simulink model "amplifierboard"  (R2020b)
settings: Solver=FixedStepDiscrete  StartTime=0.0  StopTime=2  FixedStep=0.01  RelTol=1e-3
InitFcn:
  | mbd_s32k_consistency_checks(bdroot(gcs));
undefined symbols (not defined in the file): AutoLowerVal, AutoRaiseVal, HoldVal, LED_En, LED_Off, LED_On, Logic_High, Logic_Low, LQFP, ManualLowerVal, ManualRaiseVal, PWRWNDW_CHDLCK, sC_bool_PWMEN, sC_cnt_FWSetting, sC_cnt_Mtr_DrvNo_HB, sC_cnt_PWMHB1to4, sC_cnt_PWMHB5to8, sC_cnt_TargetSlowRange, sC_pct_ManualMax, sC_pct_RampDwn, sC_pct_RampUp, sC_pct_StartPWM, sC_pct_Targetmax, SwitchPackRangeOffset, Threshold_Value, Tolerant_Time
libraries: mbd_s32k1xx_ec_toolbox x205, simulink x59, canmsglib x19, Filter x15, wndwcmd x3
(part 1 of 6)
settings Model: Creator=ur013317  LastModifiedBy=paulstu3
settings DataIOCC: ExternalInput=off  InitialState=off  SaveOutput=off  SignalLogging=off  SaveTime=off
settings OptimizationCC: DefaultParameterBehavior=Inlined  StrengthReduction=on  PassReuseOutputArgsAs=Individual arguments  ZeroExternalMemoryAtStartup=off  ZeroInternalMemoryAtStartup=off  OptimizeBlockOrder=speed  OptimizationPriority=Speed  OptimizationCustomize=off  MultiThreadedLoops=on  EfficientTunableParamExpr=on
settings DebuggingCC: InheritedTsInSrcMsg=none  SingleTaskRateTransMsg=error  ParameterTunabilityLossMsg=error  UnconnectedInputMsg=error  UnconnectedOutputMsg=error  UnconnectedLineMsg=error  UnknownTsInhSupMsg=error
settings HardwareCC: ProdBitPerPointer=32  ProdBitPerSizeT=32  ProdBitPerPtrDiffT=32  ProdLargestAtomicInteger=Long  ProdLargestAtomicFloat=Double  ProdWordSize=32  ProdHWDeviceType=ARM Compatible->ARM Cortex
settings SFSimCC: MATLABDynamicMemAlloc=off
settings RTWCC: Description=Model Based Design Toolbox S32K1xx Code Generation Target  SystemTargetFile=mbd_s32k.tlc  MakeCommand=mbd_s32k_make_rtw COPY_MDLREF_INCLUDES=0  TemplateMakefile=mbd_s32k.tmf  GenerateReport=on  IncludeHyperlinkInReport=on  LaunchReport=on  GenerateTraceInfo=on  GenerateTraceReport=on  GenerateTraceReportSl=on  GenerateTraceReportSf=on  GenerateTraceReportEml=on  CheckMdlBeforeBuild=Warning
settings CodeAppCC: ForceParamTrailComments=on  IgnoreCustomStorageClasses=off  OperatorAnnotations=on  SimulinkDataObjDesc=on  SFDataObjDesc=on  InsertBlockDesc=on
settings STFCustomTargetCC: TargetLangStandard=C99 (ISO)  MultiwordLength=256  ConcurrentExecutionCompliant=off  CombineOutputUpdateFcns=on  ERTCustomFileBanners=on  SupportContinuousTime=off  SupportNonInlinedSFcns=off  RemoveResetFunc=on  MATLABClassNameForMDSCustomization=Simulink.SoftwareTarget.ERTCustomization  CPPClassGenCompliant=off  GRTInterface=off  SystemTargetFile=mbd_s32k.tlc
settings ERTTargetCC: TargetLangStandard=C99 (ISO)  ParMdlRefBuildCompliant=off  CompOptLevelCompliant=off  ConcurrentExecutionCompliant=off  ModelStepFunctionPrototypeControlCompliant=off  CPPClassGenCompliant=off  UseToolchainInfoCompliant=off  InlinedParameterPlacement=NonHierarchical  ERTSrcFileBannerTemplate=mbd_ert_code_template.cgt  ERTHdrFileBannerTemplate=mbd_ert_code_template.cgt  ERTDataSrcFileTemplate=mbd_ert_code_template.cgt  ERTDataHdrFileTemplate=mbd_ert_code_template.cgt  ERTCustomFileTemplate=example_file_process.tlc

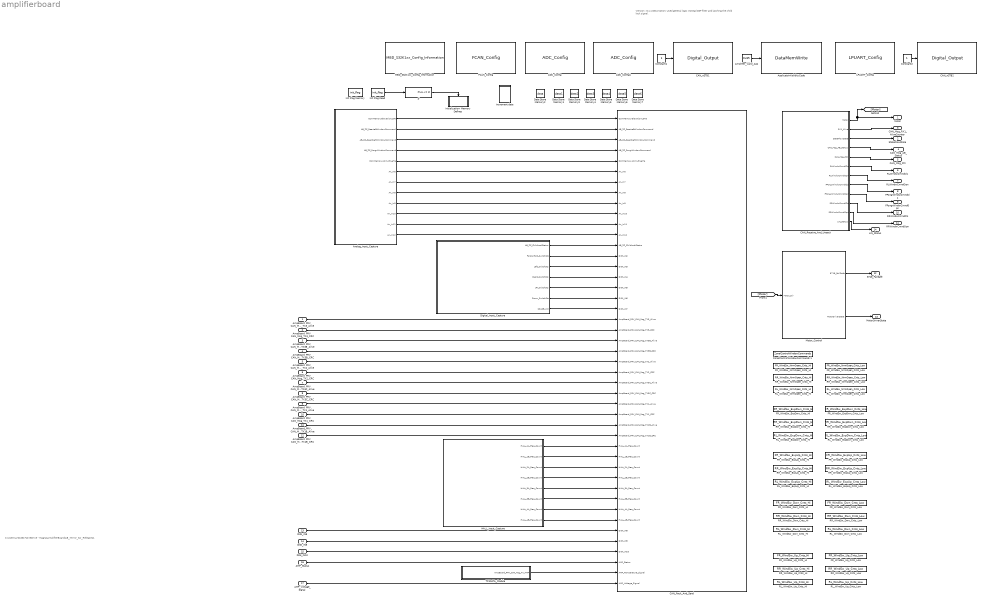
== system amplifierboard ==
  note: C:\Users\ur013317\OneDrive - Magna\AmplifierBoard\AB_Mirror_Sw_Release11
  note: Version : 6.1.1
      | Description:
      | Used general logic instead DSP filter and latching the child lock signal.
  AmpBoard_PRV_CAN_Msg_TX3_Alive : Inport
  AmpBoard_PRV_CAN_Msg_TX3_CRC : Inport  Port=2
  AmpBoard_PRV_CAN_Msg_TX3B_Alive : Inport  Port=3
  AmpBoard_PRV_CAN_Msg_TX3B_CRC : Inport  Port=4
  AmpBoard_PRV_CAN_Msg_TX2_Alive : Inport  Port=5
  AmpBoard_PRV_CAN_Msg_TX2_CRC : Inport  Port=6
  AmpBoard_PRV_CAN_Msg_TX3C_Alive : Inport  Port=7
  AmpBoard_PRV_CAN_Msg_TX3C_CRC : Inport  Port=8
  AmpBoard_PRV_CAN_Msg_TX1_Alive : Inport  Port=9
  AmpBoard_PRV_CAN_Msg_TX1_CRC : Inport  Port=10
  AmpBoard_PRV_CAN_Msg_TX1B_Alive : Inport  Port=11
  AmpBoard_PRV_CAN_Msg_TX1B_CRC : Inport  Port=12
  DIGI_IN8 : Inport  Port=13
  DIGI_IN9 : Inport  Port=14
  DIGI_IN10 : Inport  Port=15
  AMP_Status : Inport  Port=16
  AMP_Voltage_SIgnal : Inport  Port=17
  ADC_Config : mbd_s32k1xx_ec_toolbox/Motor Control Blocks/ADC Blocks/ADC_Config  instance=1  mode=12-bit conversion  smplts=2  adiclk=alternate clock 1  adiv=input clock  show_adv_opts=off  pretrgsel=PDB pre-trigger  swpretrg=Disabled  adtrg=software  trgsel=TRGMUX output  refsel=Vrefh and Vrefl  supply_monitoring=off  acfe=off  acfgt=off  acren=off  cv1=0  cv2=0  adco=off  avge=off  avgs=4 samples
  ADC_Config1 : mbd_s32k1xx_ec_toolbox/Motor Control Blocks/ADC Blocks/ADC_Config  instance=0  mode=12-bit conversion  smplts=2  adiclk=alternate clock 1  adiv=input clock  show_adv_opts=off  pretrgsel=PDB pre-trigger  swpretrg=Disabled  adtrg=software  trgsel=TRGMUX output  refsel=Vrefh and Vrefl  supply_monitoring=off  acfe=off  acfgt=off  acren=off  cv1=0  cv2=0  adco=off  avge=off  avgs=4 samples
  Amplifier_Valid_App : Constant  Value=0x85  OutDataTypeStr=uint8
  Analog_Input_Capture : Subsystem
  ApplicatoinValidityCode : mbd_s32k1xx_ec_toolbox/Utility Blocks/DataMemWrite  Priority=15  base=0x14000000  offset=0x0000  ptr=uint8_t
  CAN_Pack_And_Send : Subsystem
  CAN_Receive_And_Unpack : Subsystem
  CAN_nSTB1 : mbd_s32k1xx_ec_toolbox/GPIO Blocks/Digital_Output  gpio_pin=PTE3: [PTE3 | Port E I/O]  init_val=High  drive_strength=High
  CAN_nSTB2 : mbd_s32k1xx_ec_toolbox/GPIO Blocks/Digital_Output  gpio_pin=PTD11: [PTD11 | Port D I/O]  init_val=High  drive_strength=High
  Constant1 : Constant  OutDataTypeStr=boolean
  Constant2 : Constant  OutDataTypeStr=boolean
  Data Store Memory1 : DataStoreMemory  DataStoreName=data1  ReadBeforeWriteMsg=warning  WriteAfterWriteMsg=warning  WriteAfterReadMsg=warning  ShowAdditionalParam=off
  Data Store Memory2 : DataStoreMemory  DataStoreName=data  ReadBeforeWriteMsg=warning  WriteAfterWriteMsg=warning  WriteAfterReadMsg=warning  ShowAdditionalParam=off
  Data Store Memory3 : DataStoreMemory  DataStoreName=data2  ReadBeforeWriteMsg=warning  WriteAfterWriteMsg=warning  WriteAfterReadMsg=warning  ShowAdditionalParam=off
  Data Store Memory4 : DataStoreMemory  DataStoreName=data3  ReadBeforeWriteMsg=warning  WriteAfterWriteMsg=warning  WriteAfterReadMsg=warning  ShowAdditionalParam=off
  Data Store Memory5 : DataStoreMemory  DataStoreName=data4  ReadBeforeWriteMsg=warning  WriteAfterWriteMsg=warning  WriteAfterReadMsg=warning  ShowAdditionalParam=off
  Data Store Memory6 : DataStoreMemory  DataStoreName=data5  ReadBeforeWriteMsg=warning  WriteAfterWriteMsg=warning  WriteAfterReadMsg=warning  ShowAdditionalParam=off
  Data Store Memory7 : DataStoreMemory  DataStoreName=data6  ReadBeforeWriteMsg=warning  WriteAfterWriteMsg=warning  WriteAfterReadMsg=warning  ShowAdditionalParam=off
  Digital_Input_Capture : Subsystem
  FCAN_Config : mbd_s32k1xx_ec_toolbox/Communication Blocks/CAN Blocks/FCAN_Config  Priority=1  can_instance=1  can_mode=Normal mode  can_max_num_mb=32  can_rx=PTC6: [CAN1_RX | CAN Rx channel]  can_tx=PTC7: [CAN1_TX | CAN Tx Channel]  show_adv_opts=on  can_clk_src=Peripheral clock  can_clk_freq=80 MHz  bitrate_to_time_seg=on  bitrate=500  sample_point=87.5  real_bitrate=500  real_sample_point=87.5  prop_delay=250  bus_length=1  tq=125.0  time_quanta=16  can_presdiv=10  can_propseg=5  can_pseg1=8  can_pseg2=2  can_rjw=2  cbt_bitrate=2000  cbt_sample_point=80  cbt_real_bitrate=2000  cbt_real_sample_point=80  cbt_tq=25.0  cbt_time_quanta=40  can_cbt_presdiv=4  can_cbt_propseg=9  can_cbt_pseg1=5  can_cbt_pseg2=5  can_cbt_rjw=3  can_fd_enable=off  can_payload=8  tdc_enable=off  tdc_offset=20  can_rxfifo_enable=off  can_num_id_filters=8  can_fifo_id_format=A  can_fifo_id_filter={{false,false,'0x2'},{false,false,'0x3'},{false,false,'0x4'},{false,false,'0xAB'},{false,false,'0x0'},{false,false,'0x0'},{false,false,'0x0'},{false,false,'0x0'}}  can_pn_enable=off  can_wakeup_match=off  can_wakeup_timeout=off  can_timeout_en=off  can_match_timeout=1  can_multiple_matches_en=off  can_num_matches=1  can_idfilter_extendedid=off  can_idfilter_remoteframe=off  can_idfilter_type=Match exact  can_idfilter_id1=0  can_idfilter_id2=0  can_payloadfilter_enable=off  can_payloadfilter_dlclow=0  can_payloadfilter_dlchigh=0  can_payloadfilter_type=Match exact  can_payloadfilter_payload1_b0=0  can_payloadfilter_payload1_b1=0  can_payloadfilter_payload1_b2=0  can_payloadfilter_payload1_b3=0  can_payloadfilter_payload1_b4=0  can_payloadfilter_payload1_b5=0  can_payloadfilter_payload1_b6=0  can_payloadfilter_payload1_b7=0  can_payloadfilter_payload2_b0=0  can_payloadfilter_payload2_b1=0  can_payloadfilter_payload2_b2=0  can_payloadfilter_payload2_b3=0  can_payloadfilter_payload2_b4=0  can_payloadfilter_payload2_b5=0  can_payloadfilter_payload2_b6=0  can_payloadfilter_payload2_b7=0
  FR_WindSw_Dwn_Cnts_Hi : DataStoreMemory  DataStoreName=FR_WindSw_Dwn_Cnts_Hi  ReadBeforeWriteMsg=warning  WriteAfterWriteMsg=warning  WriteAfterReadMsg=warning  ShowAdditionalParam=off  OutDataTypeStr=uint16
  FR_WindSw_Dwn_Cnts_Low : DataStoreMemory  DataStoreName=FR_WindSw_Dwn_Cnts_Low  ReadBeforeWriteMsg=warning  WriteAfterWriteMsg=warning  WriteAfterReadMsg=warning  ShowAdditionalParam=off  OutDataTypeStr=uint16
  FR_WindSw_ExpDwn_Cnts_Hi : DataStoreMemory  DataStoreName=FR_WindSw_ExpDwn_Cnts_Hi  ReadBeforeWriteMsg=warning  WriteAfterWriteMsg=warning  WriteAfterReadMsg=warning  ShowAdditionalParam=off  OutDataTypeStr=uint16
  FR_WindSw_ExpDwn_Cnts_Low : DataStoreMemory  DataStoreName=FR_WindSw_ExpDwn_Cnts_Low  ReadBeforeWriteMsg=warning  WriteAfterWriteMsg=warning  WriteAfterReadMsg=warning  ShowAdditionalParam=off  OutDataTypeStr=uint16
  FR_WindSw_ExpUp_Cnts_Hi : DataStoreMemory  DataStoreName=FR_WindSw_ExpUp_Cnts_Hi  ReadBeforeWriteMsg=warning  WriteAfterWriteMsg=warning  WriteAfterReadMsg=warning  ShowAdditionalParam=off  OutDataTypeStr=uint16
  FR_WindSw_ExpUp_Cnts_Low : DataStoreMemory  DataStoreName=FR_WindSw_ExpUp_Cnts_Low  ReadBeforeWriteMsg=warning  WriteAfterWriteMsg=warning  WriteAfterReadMsg=warning  ShowAdditionalParam=off  OutDataTypeStr=uint16
  "FR_WindSw_NrmOpen_Cnts_Hi " : DataStoreMemory  DataStoreName=FR_WindSw_NrmOpen_Cnts_Hi  ReadBeforeWriteMsg=warning  WriteAfterWriteMsg=warning  WriteAfterReadMsg=warning  ShowAdditionalParam=off  OutDataTypeStr=uint16
  FR_WindSw_NrmOpen_Cnts_Low : DataStoreMemory  DataStoreName=FR_WindSw_NrmOpen_Cnts_Low  ReadBeforeWriteMsg=warning  WriteAfterWriteMsg=warning  WriteAfterReadMsg=warning  ShowAdditionalParam=off  OutDataTypeStr=uint16
  FR_WindSw_Up_Cnts_Hi : DataStoreMemory  DataStoreName=FR_WindSw_Up_Cnts_Hi  ReadBeforeWriteMsg=warning  WriteAfterWriteMsg=warning  WriteAfterReadMsg=warning  ShowAdditionalParam=off  OutDataTypeStr=uint16
      settings: LockScale=on
  FR_WindSw_Up_Cnts_Low : DataStoreMemory  DataStoreName=FR_WindSw_Up_Cnts_Low  ReadBeforeWriteMsg=warning  WriteAfterWriteMsg=warning  WriteAfterReadMsg=warning  ShowAdditionalParam=off  OutDataTypeStr=uint16
  HALL_Input_Capture : Subsystem
  If : If  IfExpression=u1 <= 2  ShowElse=off
  Increment data : Subsystem
  Init Flag Memory : DataStoreMemory  DataStoreName=init_flag  ReadBeforeWriteMsg=warning  WriteAfterWriteMsg=warning  WriteAfterReadMsg=warning  ShowAdditionalParam=off  OutDataTypeStr=fixdt('uint8', 'DataTypeOverride', 'Off')
  Init Flag Read : DataStoreRead  DataStoreName=init_flag  DataStoreElements=init_flag
  Initialization- Memory Defines : Subsystem  TreatAsAtomicUnit=on
  LPUART_Config : mbd_s32k1xx_ec_toolbox/Communication Blocks/UART Blocks/LPUART_Config  instance=2  baudrate=115200  custom_baudrate=1000000  databits=8  parity=None  sbns=1  bothedge=rising edge  rxinv=off  txinv=off  show_adv_opts=off  brk13=10 - 13 bit times  lbkde=10 - 13 bit times  rx=PTD6: [LPUART2_RX | Receive]  tx=PTD7: [LPUART2_TX | Transmit]
  MBD_S32K1xx_Config_Information : mbd_s32k1xx_ec_toolbox/MBD_S32K1xx_Config_Information  Priority=2  mbdt_ver=0  disp_str=|  config_params=[]  mcu_target_name=S32K146  mcu_target_package=100-LQFP  mcu_target_sram_size=128KB  mcu_system_clock_freq=80  mcu_xtal_freq=External 40  mcu_steptick_timer=LPIT Channel 0  mcu_steptick_prio=15  ds_import_enable=on  target_compiler=GCC  target_memory=FLASH  gcc_target_compile_opts=-mthumb -mfloat-abi=hard -mfpu=fpv4-sp-d16 -O1 -g -gstrict-dwarf  gcc_target_assemble_opts=-mthumb -mfloat-abi=hard -mfpu=fpv4-sp-d16 -g  gcc_target_link_opts=-mthumb -mfloat-abi=hard -mfpu=fpv4-sp-d16  gcc_target_default_lcf=off  gcc_target_user_lcf=S32K146_128_flash.ld  ghs_target_compile_opts=-cpu=cortexm4f -thumb -fpu=vfpv4_d16 -fsingle -Ogeneral -Wundef -Wimplicit-int -Wshadow -Wtrigraphs --no_commons --gnu_asm -gnu99 -gdwarf-2 -G  ghs_target_assemble_opts=-cpu=cortexm4f -fpu=vfpv4_d16  ghs_target_link_opts=-cpu=cortexm4f -thumb -fpu=vfpv4_d16  ghs_target_default_lcf=on  ghs_target_user_lcf=S32K146_128_flash.ld  iar_target_compile_opts=--cpu=Cortex-M4F --thumb --fpu=VFPv4_sp -Ol -e --debug --dlib_config normal  iar_target_assemble_opts=--cpu Cortex-M4F --thumb --fpu VFPv4_sp  iar_target_link_opts=--no_exceptions --vfe --inline  iar_target_default_lcf=on  iar_target_user_lcf=S32K146_128_flash.icf  pil_download_enable=off  rbl_download_enable=on  rbl_start_delay=5000  rbl_download_interface=OpenSDA  rbl_restart_request=off  rbl_com_port=Custom  rbl_com_port_custom=COM1  pil_download_rate=57600  pil_download_rate_custom=115200  pil_opensda_drive=Custom  pil_opensda_drive_custom=D  jtag_interface=OpenSDA Embedded Debug  jlink_default_path=on  jlink_user_path=C:\Program Files\SEGGER\JLink\  pil_uart_instance=1  pil_uart_rx=PTC6: [LPUART1_RX | Receive]  pil_uart_tx=PTC7: [LPUART1_TX | Transmit]  FTM_PWM_PcrCheckEnDis=on  FTM_Input_Edge_Inputs_PcrCheckEnDis=on  FTM_Dual_Edge_Inputs_PcrCheckEnDis=on  FTM_Quadrature_Inputs_PcrCheckEnDis=on  FTM_Hall_Sensor_Inputs_PcrCheckEnDis=on  LPTMR_PcrCheckEnDis=on  PIT_PcrCheckEnDis=on  RTC_PcrCheckEnDis=on  FlexCAN_PcrCheckEnDis=on  LIN_PcrCheckEnDis=on  FlexIO_PcrCheckEnDis=on  LPI2C_PcrCheckEnDis=on  LPSPI_PcrCheckEnDis=on  LPUART_PcrCheckEnDis=on  CMP_PcrCheckEnDis=on  GPIO_OutputPcrCheckEnDis=on  GPIO_InputPcrCheckEnDis=on  SBC_PcrCheckEnDis=on  BMS_PcrCheckEnDis=on  AMMCLIB_PcrCheckEnDis=on  FM_PcrCheckEnDis=on  Profile_PcrCheckEnDis=on  ConfigParams_PcrCheckEnDis=on  ModelRef_PcrCheckEnDis=on  PDB0_PcrCheckEnDis=on  CSEc_PcrCheckEnDis=on  eDMA_PcrCheckEnDis=on  FLASH_PcrCheckEnDis=on  ADC_PcrCheckEnDis=on  WDOG_PcrCheckEnDis=on
      | Target : S32K144-64KB_SRAM
      | Package : 100-pin
      | System clock : 80 MHz
      | XTAL clock : External 8 MHz
      | Compiler : IAR
      | Target Type : FLASH
      | Download Code after build : off
      | Step Tick Interrupt Priority : 15
  Motor_Control : Subsystem
  RL_WindSw_Dwn_Cnts_Hi : DataStoreMemory  DataStoreName=RL_WindSw_Dwn_Cnts_Hi  ReadBeforeWriteMsg=warning  WriteAfterWriteMsg=warning  WriteAfterReadMsg=warning  ShowAdditionalParam=off  OutDataTypeStr=uint16
  RL_WindSw_Dwn_Cnts_Low : DataStoreMemory  DataStoreName=RL_WindSw_Dwn_Cnts_Low  ReadBeforeWriteMsg=warning  WriteAfterWriteMsg=warning  WriteAfterReadMsg=warning  ShowAdditionalParam=off  OutDataTypeStr=uint16
  RL_WindSw_ExpDwn_Cnts_Hi : DataStoreMemory  DataStoreName=RL_WindSw_ExpDwn_Cnts_Hi  ReadBeforeWriteMsg=warning  WriteAfterWriteMsg=warning  WriteAfterReadMsg=warning  ShowAdditionalParam=off  OutDataTypeStr=uint16
  RL_WindSw_ExpDwn_Cnts_Low : DataStoreMemory  DataStoreName=RL_WindSw_ExpDwn_Cnts_Low  ReadBeforeWriteMsg=warning  WriteAfterWriteMsg=warning  WriteAfterReadMsg=warning  ShowAdditionalParam=off  OutDataTypeStr=uint16
  RL_WindSw_ExpUp_Cnts_Hi : DataStoreMemory  DataStoreName=RL_WindSw_ExpUp_Cnts_Hi  ReadBeforeWriteMsg=warning  WriteAfterWriteMsg=warning  WriteAfterReadMsg=warning  ShowAdditionalParam=off  OutDataTypeStr=uint16
  RL_WindSw_ExpUp_Cnts_Low : DataStoreMemory  DataStoreName=RL_WindSw_ExpUp_Cnts_Low  ReadBeforeWriteMsg=warning  WriteAfterWriteMsg=warning  WriteAfterReadMsg=warning  ShowAdditionalParam=off  OutDataTypeStr=uint16
  RL_WindSw_NrmOpen_Cnts_Hi : DataStoreMemory  DataStoreName=RL_WindSw_NrmOpen_Cnts_Hi  ReadBeforeWriteMsg=warning  WriteAfterWriteMsg=warning  WriteAfterReadMsg=warning  ShowAdditionalParam=off  OutDataTypeStr=uint16
  RL_WindSw_NrmOpen_Cnts_Low : DataStoreMemory  DataStoreName=RL_WindSw_NrmOpen_Cnts_Low  ReadBeforeWriteMsg=warning  WriteAfterWriteMsg=warning  WriteAfterReadMsg=warning  ShowAdditionalParam=off  OutDataTypeStr=uint16
  RL_WindSw_Up_Cnts_Hi : DataStoreMemory  DataStoreName=RL_WindSw_Up_Cnts_Hi  ReadBeforeWriteMsg=warning  WriteAfterWriteMsg=warning  WriteAfterReadMsg=warning  ShowAdditionalParam=off  OutDataTypeStr=uint16
  RL_WindSw_Up_Cnts_Low : DataStoreMemory  DataStoreName=RL_WindSw_Up_Cnts_Low  ReadBeforeWriteMsg=warning  WriteAfterWriteMsg=warning  WriteAfterReadMsg=warning  ShowAdditionalParam=off  OutDataTypeStr=uint16
  RR_WindSw_Dwn_Cnts_Hi : DataStoreMemory  DataStoreName=RR_WindSw_Dwn_Cnts_Hi  ReadBeforeWriteMsg=warning  WriteAfterWriteMsg=warning  WriteAfterReadMsg=warning  ShowAdditionalParam=off  OutDataTypeStr=uint16
  RR_WindSw_Dwn_Cnts_Low : DataStoreMemory  DataStoreName=RR_WindSw_Dwn_Cnts_Low  ReadBeforeWriteMsg=warning  WriteAfterWriteMsg=warning  WriteAfterReadMsg=warning  ShowAdditionalParam=off  OutDataTypeStr=uint16
  RR_WindSw_ExpDwn_Cnts_Hi : DataStoreMemory  DataStoreName=RR_WindSw_ExpDwn_Cnts_Hi  ReadBeforeWriteMsg=warning  WriteAfterWriteMsg=warning  WriteAfterReadMsg=warning  ShowAdditionalParam=off  OutDataTypeStr=uint16
  RR_WindSw_ExpDwn_Cnts_Low : DataStoreMemory  DataStoreName=RR_WindSw_ExpDwn_Cnts_Low  ReadBeforeWriteMsg=warning  WriteAfterWriteMsg=warning  WriteAfterReadMsg=warning  ShowAdditionalParam=off  OutDataTypeStr=uint16
  RR_WindSw_ExpUp_Cnts_Hi : DataStoreMemory  DataStoreName=RR_WindSw_ExpUp_Cnts_Hi  ReadBeforeWriteMsg=warning  WriteAfterWriteMsg=warning  WriteAfterReadMsg=warning  ShowAdditionalParam=off  OutDataTypeStr=uint16
  RR_WindSw_ExpUp_Cnts_Low : DataStoreMemory  DataStoreName=RR_WindSw_ExpUp_Cnts_Low  ReadBeforeWriteMsg=warning  WriteAfterWriteMsg=warning  WriteAfterReadMsg=warning  ShowAdditionalParam=off  OutDataTypeStr=uint16
  RR_WindSw_NrmOpen_Cnts_Hi : DataStoreMemory  DataStoreName=RR_WindSw_NrmOpen_Cnts_Hi  ReadBeforeWriteMsg=warning  WriteAfterWriteMsg=warning  WriteAfterReadMsg=warning  ShowAdditionalParam=off  OutDataTypeStr=uint16
  RR_WindSw_NrmOpen_Cnts_Low : DataStoreMemory  DataStoreName=RR_WindSw_NrmOpen_Cnts_Low  ReadBeforeWriteMsg=warning  WriteAfterWriteMsg=warning  WriteAfterReadMsg=warning  ShowAdditionalParam=off  OutDataTypeStr=uint16
  RR_WindSw_Up_Cnts_Hi : DataStoreMemory  DataStoreName=RR_WindSw_Up_Cnts_Hi  ReadBeforeWriteMsg=warning  WriteAfterWriteMsg=warning  WriteAfterReadMsg=warning  ShowAdditionalParam=off  OutDataTypeStr=uint16
  RR_WindSw_Up_Cnts_Low : DataStoreMemory  DataStoreName=RR_WindSw_Up_Cnts_Low  ReadBeforeWriteMsg=warning  WriteAfterWriteMsg=warning  WriteAfterReadMsg=warning  ShowAdditionalParam=off  OutDataTypeStr=uint16
  TC1047A_Module : Subsystem
  ZonalControlWindowCommands 1 : DataStoreMemory  DataStoreName=ZonalControlWindowCommands  ReadBeforeWriteMsg=warning  WriteAfterWriteMsg=warning  WriteAfterReadMsg=warning  ShowAdditionalParam=off  OutDataTypeStr=uint16
  Motor : Outport
  StateFlowState : Outport  Port=2
  CHN_Msg_RX1_AliveCounter : Outport  Port=3
  CAN_Msg_AB_Status : Outport  Port=4
  CAN_Msg_PCI : Outport  Port=5
  RLWindwCmndCls : Outport  Port=6
  RLWindwCmndOpn : Outport  Port=7
  FPsngrWindwCmndCls : Outport  Port=8
  FPsngrWindwCmndOpn : Outport  Port=9
  RRWindwCmndCls : Outport  Port=10
  RRWindwCmndOpn : Outport  Port=11
  8718_FailSafe : Outport  Port=12
  MotorDriverState : Outport  Port=13
  LIN_Status : Outport  Port=14
  wires:
  Constant1/1 -> CAN_nSTB1/1
  If/1 -> Initialization- Memory Defines/Action
  Init Flag Read/1 -> If/1
  [Motor] -> Motor_Control/1(Motor_Dir)
  Analog_Input_Capture/6(An_In6) -> CAN_Pack_And_Send/6(An_In6)
  Analog_Input_Capture/7(An_In7) -> CAN_Pack_And_Send/7(An_In7)
  Analog_Input_Capture/8(An_In8) -> CAN_Pack_And_Send/8(An_In8)
  Analog_Input_Capture/9(An_In9) -> CAN_Pack_And_Send/9(An_In9)
  Analog_Input_Capture/10(An_In10) -> CAN_Pack_And_Send/10(An_In10)
  Analog_Input_Capture/11(An_In11) -> CAN_Pack_And_Send/11(An_In11)
  Analog_Input_Capture/12(An_In12) -> CAN_Pack_And_Send/12(An_In12)
  Digital_Input_Capture/2(FoldUnfold_SwitchSts) -> CAN_Pack_And_Send/14(DIGI_IN2)
  Digital_Input_Capture/3(Left_SwitchSts) -> CAN_Pack_And_Send/15(DIGI_IN3)
  Digital_Input_Capture/4(Right_SwitchSts) -> CAN_Pack_And_Send/16(DIGI_IN4)
  Digital_Input_Capture/5(UP_SwitchSts) -> CAN_Pack_And_Send/17(DIGI_IN5)
  Digital_Input_Capture/6(Down_SwitchSts) -> CAN_Pack_And_Send/18(DIGI_IN6)
  Digital_Input_Capture/7(SPARE_In3) -> CAN_Pack_And_Send/19(DIGI_IN7)
  AmpBoard_PRV_CAN_Msg_TX3_Alive/1 -> CAN_Pack_And_Send/20(AmpBoard_PRV_CAN_Msg_TX3_Alive)
  AmpBoard_PRV_CAN_Msg_TX3_CRC/1 -> CAN_Pack_And_Send/21(AmpBoard_PRV_CAN_Msg_TX3_CRC)
  AmpBoard_PRV_CAN_Msg_TX3B_Alive/1 -> CAN_Pack_And_Send/22(AmpBoard_PRV_CAN_Msg_TX3B_Alive)
  AmpBoard_PRV_CAN_Msg_TX3B_CRC/1 -> CAN_Pack_And_Send/23(AmpBoard_PRV_CAN_Msg_TX3B_CRC)
  AmpBoard_PRV_CAN_Msg_TX2_Alive/1 -> CAN_Pack_And_Send/24(AmpBoard_PRV_CAN_Msg_TX2_Alive)
  AmpBoard_PRV_CAN_Msg_TX2_CRC/1 -> CAN_Pack_And_Send/25(AmpBoard_PRV_CAN_Msg_TX2_CRC)
  AmpBoard_PRV_CAN_Msg_TX3C_Alive/1 -> CAN_Pack_And_Send/26(AmpBoard_PRV_CAN_Msg_TX3C_Alive)
  AmpBoard_PRV_CAN_Msg_TX3C_CRC/1 -> CAN_Pack_And_Send/27(AmpBoard_PRV_CAN_Msg_TX3C_CRC)
  AmpBoard_PRV_CAN_Msg_TX1_Alive/1 -> CAN_Pack_And_Send/28(AmpBoard_PRV_CAN_Msg_TX1_Alive)
  AmpBoard_PRV_CAN_Msg_TX1_CRC/1 -> CAN_Pack_And_Send/29(AmpBoard_PRV_CAN_Msg_TX1_CRC)
  AmpBoard_PRV_CAN_Msg_TX1B_Alive/1 -> CAN_Pack_And_Send/30(AmpBoard_PRV_CAN_Msg_TX1B_Alive)
  AmpBoard_PRV_CAN_Msg_TX1B_CRC/1 -> CAN_Pack_And_Send/31(AmpBoard_PRV_CAN_Msg_TX1B_CRC)
  HALL_Input_Capture/1(HALL_1A_Freq_Count) -> CAN_Pack_And_Send/32(HALL_1A_Freq_Count)
  HALL_Input_Capture/2(HALL_1B_Freq_Count) -> CAN_Pack_And_Send/33(HALL_1B_Freq_Count)
  HALL_Input_Capture/3(HALL_2A_Freq_Count) -> CAN_Pack_And_Send/34(HALL_2A_Freq_Count)
  HALL_Input_Capture/4(HALL_2B_Freq_Count) -> CAN_Pack_And_Send/35(HALL_2B_Freq_Count)
  HALL_Input_Capture/5(HALL_3A_Freq_Count) -> CAN_Pack_And_Send/36(HALL_3A_Freq_Count)
  HALL_Input_Capture/6(HALL_3B_Freq_Count) -> CAN_Pack_And_Send/37(HALL_3B_Freq_Count)
  HALL_Input_Capture/7(HALL_4A_Freq_Count) -> CAN_Pack_And_Send/38(HALL_4A_Freq_Count)
  HALL_Input_Capture/8(HALL_4B_Freq_Count) -> CAN_Pack_And_Send/39(HALL_4B_Freq_Count)
  Analog_Input_Capture/1(OsmMemoryElevationLeHa) -> CAN_Pack_And_Send/1(OsmMemoryElevationLeHa)
  DIGI_IN9/1 -> CAN_Pack_And_Send/41(DIGI_IN9)
  DIGI_IN8/1 -> CAN_Pack_And_Send/40(DIGI_IN8)
  DIGI_IN10/1 -> CAN_Pack_And_Send/42(DIGI_IN10)
  Digital_Input_Capture/1(AB_ZC_ChildLockStatus) -> CAN_Pack_And_Send/13(AB_ZC_ChildLockStatus)
  Analog_Input_Capture/5(OsmMemoryAzimuthLeHa) -> CAN_Pack_And_Send/5(OsmMemoryAzimuthLeHa)
  Analog_Input_Capture/4(AB_ZC_PsngrWindowCommand) -> CAN_Pack_And_Send/4(AB_ZC_PsngrWindowCommand)
  AMP_Voltage_SIgnal/1 -> CAN_Pack_And_Send/45(AMP_Voltage_SIgnal)
  TC1047A_Module/1(AmpBoard_PRV_CAN_Msg_TX_TMP) -> CAN_Pack_And_Send/44(AMP_Temperature_Signal)
  AMP_Status/1 -> CAN_Pack_And_Send/43(AMP_Status)
  Amplifier_Valid_App/1 -> ApplicatoinValidityCode/1
  Analog_Input_Capture/2(AB_ZC_RearLeftWindowCommand) -> CAN_Pack_And_Send/2(AB_ZC_RearLeftWindowCommand)
  Analog_Input_Capture/3(AB_ZC_RearRightWindowCommand) -> CAN_Pack_And_Send/3(AB_ZC_RearRightWindowCommand)
  Constant2/1 -> CAN_nSTB2/1
  CAN_Receive_And_Unpack/11(RRWindwCmndOpn) -> RRWindwCmndOpn/1
  CAN_Receive_And_Unpack/3(StateFlowState) -> StateFlowState/1
  CAN_Receive_And_Unpack/9(FPsngrWindwCmndOpn) -> FPsngrWindwCmndOpn/1
  CAN_Receive_And_Unpack/8(FPsngrWindwCmndCls) -> FPsngrWindwCmndCls/1
  CAN_Receive_And_Unpack/10(RRWindwCmndCls) -> RRWindwCmndCls/1
  CAN_Receive_And_Unpack/7(RLWindwCmndOpn) -> RLWindwCmndOpn/1
  CAN_Receive_And_Unpack/4(CAN_Msg_AB_Status) -> CAN_Msg_AB_Status/1
  CAN_Receive_And_Unpack/2(RX1_Alive) -> CHN_Msg_RX1_AliveCounter/1
  CAN_Receive_And_Unpack/5(CAN_Msg_PCI) -> CAN_Msg_PCI/1
  CAN_Receive_And_Unpack/1(Motor) -> [Motor], Motor/1
  CAN_Receive_And_Unpack/6(RLWindwCmndCls) -> RLWindwCmndCls/1
  Motor_Control/1(8718_FailSafe) -> 8718_FailSafe/1
  Motor_Control/2(MotorDriverState) -> MotorDriverState/1
  CAN_Receive_And_Unpack/12(LIN_Status) -> LIN_Status/1

== system amplifierboard/Analog_Input_Capture ==
  note: Description:- All Analog inputs(12) are captured through ADC block
  AB_ZC_PsngrWindowCommand_In : mbd_s32k1xx_ec_toolbox/Motor Control Blocks/ADC Blocks/ADC_Start  instance=0  adc_r=A  adc_chan=PTB2: [ADC0_SE6 | ADC Single Ended Input]  aien=off  mcuTargetUpdate=on
  AB_ZC_RearLeftWindowCommand_In : mbd_s32k1xx_ec_toolbox/Motor Control Blocks/ADC Blocks/ADC_Start  instance=0  adc_r=A  adc_chan=PTB0: [ADC0_SE4 | ADC Single Ended Input]  aien=off  mcuTargetUpdate=on
  AB_ZC_RearRightWindowCommand_In : mbd_s32k1xx_ec_toolbox/Motor Control Blocks/ADC Blocks/ADC_Start  instance=0  adc_r=A  adc_chan=PTB1: [ADC0_SE5 | ADC Single Ended Input]  aien=off  mcuTargetUpdate=on
  AnIn_1 : mbd_s32k1xx_ec_toolbox/Motor Control Blocks/ADC Blocks/ADC_Start  instance=0  adc_r=A  adc_chan=PTC14: [ADC0_SE12 | ADC Single Ended Input]  aien=off  mcuTargetUpdate=on
  AnIn_10 : mbd_s32k1xx_ec_toolbox/Motor Control Blocks/ADC Blocks/ADC_Start  instance=1  adc_r=A  adc_chan=PTB12: [ADC1_SE7 | ADC Single Ended Input]  aien=off  mcuTargetUpdate=on
  AnIn_11 : mbd_s32k1xx_ec_toolbox/Motor Control Blocks/ADC Blocks/ADC_Start  instance=1  adc_r=A  adc_chan=PTD4: [ADC1_SE6 | ADC Single Ended Input]  aien=off  mcuTargetUpdate=on
  AnIn_12 : mbd_s32k1xx_ec_toolbox/Motor Control Blocks/ADC Blocks/ADC_Start  instance=1  adc_r=A  adc_chan=PTD3: [ADC1_SE3 | ADC Single Ended Input]  aien=off  mcuTargetUpdate=on
  AnIn_5 : mbd_s32k1xx_ec_toolbox/Motor Control Blocks/ADC Blocks/ADC_Start  instance=0  adc_r=A  adc_chan=PTB3: [ADC0_SE7 | ADC Single Ended Input]  aien=off  mcuTargetUpdate=on
  AnIn_6 : mbd_s32k1xx_ec_toolbox/Motor Control Blocks/ADC Blocks/ADC_Start  instance=0  adc_r=A  adc_chan=PTA7: [ADC0_SE3 | ADC Single Ended Input]  aien=off  mcuTargetUpdate=on
  AnIn_7 : mbd_s32k1xx_ec_toolbox/Motor Control Blocks/ADC Blocks/ADC_Start  instance=1  adc_r=A  adc_chan=PTB15: [ADC1_SE14 | ADC Single Ended Input]  aien=off  mcuTargetUpdate=on
  AnIn_8 : mbd_s32k1xx_ec_toolbox/Motor Control Blocks/ADC Blocks/ADC_Start  instance=0  adc_r=A  adc_chan=PTB14: [ADC0_SE9 | ADC Single Ended Input]  aien=off  mcuTargetUpdate=on
  AnIn_9 : mbd_s32k1xx_ec_toolbox/Motor Control Blocks/ADC Blocks/ADC_Start  instance=1  adc_r=A  adc_chan=PTB13: [ADC1_SE8 | ADC Single Ended Input]  aien=off  mcuTargetUpdate=on
  Data Type Conversion : DataTypeConversion  OutDataTypeStr=uint16
  Data Type Conversion1 : DataTypeConversion  OutDataTypeStr=uint16
  Data Type Conversion2 : DataTypeConversion  OutDataTypeStr=uint16
  OsmMemoryElevationLeHa : Outport
  AB_ZC_RearLeftWindowCommand : Outport  Port=2
  AB_ZC_RearRightWindowCommand : Outport  Port=3
  AB_ZC_PsngrWindowCommand : Outport  Port=4
  OsmMemoryAzimuthLeHa : Outport  Port=5
  An_In6 : Outport  Port=6
  An_In7 : Outport  Port=7
  An_In8 : Outport  Port=8
  An_In9 : Outport  Port=9
  An_In10 : Outport  Port=10
  An_In11 : Outport  Port=11
  An_In12 : Outport  Port=12
  wires:
  AnIn_6/1 -> An_In6/1
  AnIn_8/1 -> An_In8/1
  AnIn_12/1 -> An_In12/1
  AnIn_10/1 -> An_In10/1
  AnIn_11/1 -> An_In11/1
  AnIn_7/1 -> An_In7/1
  AnIn_9/1 -> An_In9/1
  AB_ZC_PsngrWindowCommand_In/1 -> Data Type Conversion2/1
  AB_ZC_RearRightWindowCommand_In/1 -> Data Type Conversion1/1
  AB_ZC_RearLeftWindowCommand_In/1 -> Data Type Conversion/1
  AnIn_1/1 -> OsmMemoryAzimuthLeHa/1
  AnIn_5/1 -> OsmMemoryElevationLeHa/1
  Data Type Conversion/1 -> AB_ZC_RearLeftWindowCommand/1
  Data Type Conversion2/1 -> AB_ZC_PsngrWindowCommand/1
  Data Type Conversion1/1 -> AB_ZC_RearRightWindowCommand/1

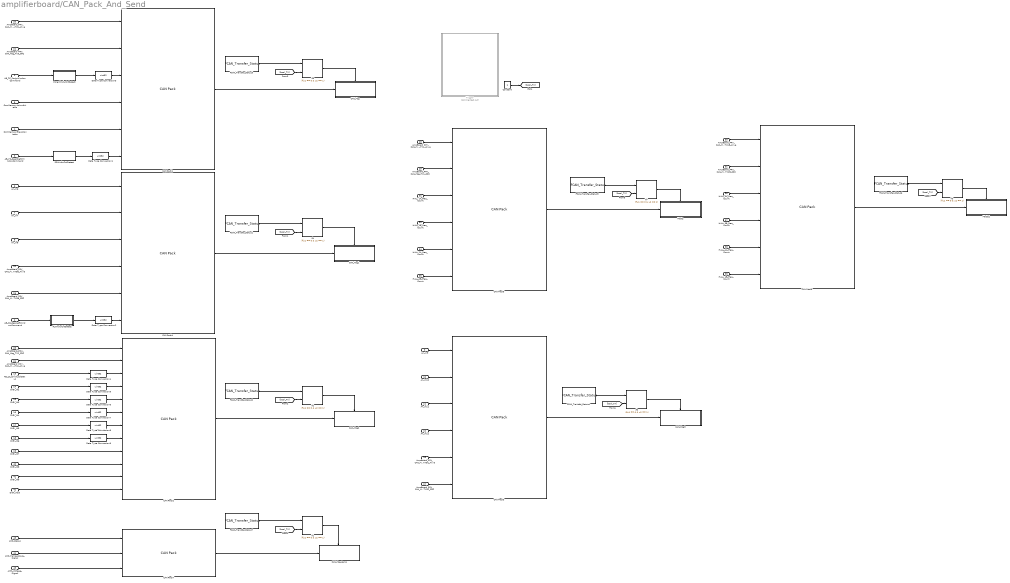
== system amplifierboard/CAN_Pack_And_Send ==
  OsmMemoryElevationLeHa : Inport
  AB_ZC_RearLeftWindowCommand : Inport  Port=2
  AB_ZC_RearRightWindowCommand : Inport  Port=3
  AB_ZC_PsngrWindowCommand : Inport  Port=4
  OsmMemoryAzimuthLeHa : Inport  Port=5
  An_In6 : Inport  Port=6
  An_In7 : Inport  Port=7
  An_In8 : Inport  Port=8
  An_In9 : Inport  Port=9
  An_In10 : Inport  Port=10
  An_In11 : Inport  Port=11
  An_In12 : Inport  Port=12
  AB_ZC_ChildLockStatus : Inport  Port=13
  DIGI_IN2 : Inport  Port=14
  DIGI_IN3 : Inport  Port=15
  DIGI_IN4 : Inport  Port=16
  DIGI_IN5 : Inport  Port=17
  DIGI_IN6 : Inport  Port=18
  DIGI_IN7 : Inport  Port=19
  AmpBoard_PRV_CAN_Msg_TX3_Alive : Inport  Port=20
  AmpBoard_PRV_CAN_Msg_TX3_CRC : Inport  Port=21
  AmpBoard_PRV_CAN_Msg_TX3B_Alive : Inport  Port=22
  AmpBoard_PRV_CAN_Msg_TX3B_CRC : Inport  Port=23
  AmpBoard_PRV_CAN_Msg_TX2_Alive : Inport  Port=24
  AmpBoard_PRV_CAN_Msg_TX2_CRC : Inport  Port=25
  AmpBoard_PRV_CAN_Msg_TX3C_Alive : Inport  Port=26
  AmpBoard_PRV_CAN_Msg_TX3C_CRC : Inport  Port=27
  AmpBoard_PRV_CAN_Msg_TX1_Alive : Inport  Port=28
  AmpBoard_PRV_CAN_Msg_TX1_CRC : Inport  Port=29
  AmpBoard_PRV_CAN_Msg_TX1B_Alive : Inport  Port=30
  AmpBoard_PRV_CAN_Msg_TX1B_CRC : Inport  Port=31
  HALL_1A_Freq_Count : Inport  Port=32
  HALL_1B_Freq_Count : Inport  Port=33
  HALL_2A_Freq_Count : Inport  Port=34
  HALL_2B_Freq_Count : Inport  Port=35
  HALL_3A_Freq_Count : Inport  Port=36
  HALL_3B_Freq_Count : Inport  Port=37
  HALL_4A_Freq_Count : Inport  Port=38
  HALL_4B_Freq_Count : Inport  Port=39
  DIGI_IN8 : Inport  Port=40
  DIGI_IN9 : Inport  Port=41
  DIGI_IN10 : Inport  Port=42
  AMP_Status : Inport  Port=43
  AMP_Temperature_Signal : Inport  Port=44
  AMP_Voltage_SIgnal : Inport  Port=45
  CAN Pack1 : canmsglib/CAN Pack  CANdbFile=C:\Work\repos\GenericAB\poc_communication_matrix\Zonal_Controller_FL\DBC_ZC_FL_CAN_3.dbc  MsgList=AB_Door_FL_PRV_CAN_Msg_TX_3  MsgName=AB_Door_FL_PRV_CAN_Msg_TX_3  MsgIDType=Standard (11-bit identifier)  MsgIdentifier=8  MsgLength=8  Remote=off  ApplyMinMax=off  BusOutput=on  SignalInfo={'AmpBoard_PRV_CAN_Msg_TX3_Alive','8','4','BE','unsigned','Standard','0','1','0','0','14';'AmpBoard_PRV_CAN_Msg_TX3_CRC','0','8','BE','unsigned','Standard','0','1','0','0','255';'FrontPsngrWindowSwitchRaw','52','12','BE','unsigned','Standard','0','1','0','0','4095';'OsmMemoryAzimuthLeHa','28','12','BE','unsigned','Standard','0','1','0','0','4095';'OsmMemoryElevationLeHa','32','12','BE','unsigned','Standard','0','1','0','0','4095';'RearRightWindowSwitchRaw','56','12','BE','unsigned','Standard','0','1','0','0','4095'}
      settings: SourceProductBaseCode=ME,XP,VN  DataFormat=CANdb specified signals
  CAN Pack2 : canmsglib/CAN Pack  CANdbFile=C:\Work\repos\GenericAB\poc_communication_matrix\Zonal_Controller_FL\DBC_ZC_FL_CAN_3.dbc  MsgList=AB_Door_FL_PRV_CAN_Msg_TX_2  MsgName=AB_Door_FL_PRV_CAN_Msg_TX_2  MsgIDType=Standard (11-bit identifier)  MsgIdentifier=7  MsgLength=8  Remote=off  ApplyMinMax=off  BusOutput=on  SignalInfo={'AmpBoard_PRV_CAN_Msg_TX2_Alive','8','4','BE','unsigned','Standard','0','1','0','0','14';'AmpBoard_PRV_CAN_Msg_TX2_CRC','0','8','BE','unsigned','Standard','0','1','0','0','255';'ChildLockSwitchRaw','16','2','LE','unsigned','Standard','0','1','0','0','3';'Switch_State_SW_02','18','2','LE','unsigned','Standard','0','1','0','0','3';'Switch_State_SW_03','20','2','LE','unsigned','Standard','0','1','0','0','3';'Switch_State_SW_04','22','2','LE','unsigned','Standard','0','1','0','0','3';'Switch_State_SW_05','24','2','LE','unsigned','Standard','0','1','0','0','3';'Switch_State_SW_06','26','2','LE','unsigned','Standard','0','1','0','0','3';'Switch_State_SW_07','28','2','LE','unsigned','Standard','0','1','0','0','3';'Switch_State_SW_08','30','2','LE','unsigned','Standard','0','1','0','0','3';'Switch_State_SW_09','32','2','LE','unsigned','Standard','0','1','0','0','3';'Switch_State_SW_10','34','2','LE','unsigned','Standard','0','1','0','0','3'}
      settings: SourceProductBaseCode=ME,XP,VN  DataFormat=CANdb specified signals
  CAN Pack3 : canmsglib/CAN Pack  CANdbFile=C:\Work\repos\GenericAB\poc_communication_matrix\Zonal_Controller_FL\DBC_ZC_FL_CAN_3.dbc  MsgList=AB_Door_FL_PRV_CAN_Msg_TX_3C  MsgName=AB_Door_FL_PRV_CAN_Msg_TX_3C  MsgIDType=Standard (11-bit identifier)  MsgIdentifier=21  MsgLength=8  Remote=off  ApplyMinMax=off  BusOutput=on  SignalInfo={'A2D_Chan_09','28','12','BE','unsigned','Standard','0','1','0','0','4095';'A2D_Chan_10','32','12','BE','unsigned','Standard','0','1','0','0','4095';'A2D_Chan_11','52','12','BE','unsigned','Standard','0','1','0','0','4095';'A2D_Chan_12','56','12','BE','unsigned','Standard','0','1','0','0','4095';'AmpBoard_PRV_CAN_Msg_TX3C_Alive','8','4','BE','unsigned','Standard','0','1','0','0','14';'AmpBoard_PRV_CAN_Msg_TX3C_CRC','0','8','BE','unsigned','Standard','0','1','0','0','255'}
      settings: SourceProductBaseCode=ME,XP,VN  DataFormat=CANdb specified signals
  CAN Pack4 : canmsglib/CAN Pack  CANdbFile=C:\Work\repos\GenericAB\poc_communication_matrix\Zonal_Controller_FL\DBC_ZC_FL_CAN_3.dbc  MsgList=AB_Door_FL_PRV_CAN_Msg_TX_3B  MsgName=AB_Door_FL_PRV_CAN_Msg_TX_3B  MsgIDType=Standard (11-bit identifier)  MsgIdentifier=19  MsgLength=8  Remote=off  ApplyMinMax=off  BusOutput=on  SignalInfo={'A2D_Chan_06','32','12','BE','unsigned','Standard','0','1','0','0','4095';'A2D_Chan_07','52','12','BE','unsigned','Standard','0','1','0','0','4095';'A2D_Chan_08','56','12','BE','unsigned','Standard','0','1','0','0','4095';'AmpBoard_PRV_CAN_Msg_TX3B_Alive','8','4','BE','unsigned','Standard','0','1','0','0','14';'AmpBoard_PRV_CAN_Msg_TX3B_CRC','0','8','BE','unsigned','Standard','0','1','0','0','255';'RearLeftWindowSwitchRaw','28','12','BE','unsigned','Standard','0','1','0','0','4095'}
      settings: SourceProductBaseCode=ME,XP,VN  DataFormat=CANdb specified signals
  CAN Pack5 : canmsglib/CAN Pack  CANdbFile=C:\Work\repos\GenericAB\poc_communication_matrix\Zonal_Controller_FL\DBC_ZC_FL_CAN_3.dbc  MsgList=AB_Door_FL_PRV_CAN_Msg_TX_1  MsgName=AB_Door_FL_PRV_CAN_Msg_TX_1  MsgIDType=Standard (11-bit identifier)  MsgIdentifier=6  MsgLength=8  Remote=off  ApplyMinMax=off  BusOutput=on  SignalInfo={'AmpBoard_PRV_CAN_Msg_TX1_Alive','8','4','BE','unsigned','Standard','0','1','0','0','14';'AmpBoard_PRV_CAN_Msg_TX1_CRC','0','8','BE','unsigned','Standard','0','1','0','0','255';'Hall_1A_Freq','30','10','BE','signed','Standard','0','1','0','-512','511';'Hall_1B_Freq','36','10','BE','signed','Standard','0','1','0','-512','511';'Hall_2A_Freq','42','10','BE','signed','Standard','0','1','0','-512','511';'Hall_2B_Freq','48','10','BE','signed','Standard','0','1','0','-512','511'}
      settings: SourceProductBaseCode=ME,XP,VN  DataFormat=CANdb specified signals
  CAN Pack6 : canmsglib/CAN Pack  CANdbFile=C:\Work\repos\GenericAB\poc_communication_matrix\Zonal_Controller_FL\DBC_ZC_FL_CAN_3.dbc  MsgList=AB_Door_FL_PRV_CAN_Msg_TX_1B  MsgName=AB_Door_FL_PRV_CAN_Msg_TX_1B  MsgIDType=Standard (11-bit identifier)  MsgIdentifier=20  MsgLength=8  Remote=off  ApplyMinMax=off  BusOutput=on  SignalInfo={'AmpBoard_PRV_CAN_Msg_TX1B_Alive','8','4','BE','unsigned','Standard','0','1','0','0','14';'AmpBoard_PRV_CAN_Msg_TX1B_CRC','0','8','BE','unsigned','Standard','0','1','0','0','255';'Hall_3A_Freq','30','10','BE','signed','Standard','0','1','0','-512','511';'Hall_3B_Freq','36','10','BE','signed','Standard','0','1','0','-512','511';'Hall_4A_Freq','42','10','BE','signed','Standard','0','1','0','-512','511';'Hall_4B_Freq','48','10','BE','signed','Standard','0','1','0','-512','511'}
      settings: SourceProductBaseCode=ME,XP,VN  DataFormat=CANdb specified signals
  CAN Pack7 : canmsglib/CAN Pack  CANdbFile=C:\Work\repos\GenericAB\poc_communication_matrix\Zonal_Controller_FL\DBC_ZC_FL_CAN_3.dbc  MsgList=AMP_Monitoring_Parameter  MsgName=AMP_Monitoring_Parameter  MsgIDType=Standard (11-bit identifier)  MsgIdentifier=275  MsgLength=8  Remote=off  ApplyMinMax=off  BusOutput=on  SignalInfo={'AMP_Status','16','8','LE','unsigned','Standard','0','1','0','0','255';'AMP_Temperature_Signal','24','16','LE','unsigned','Standard','0','0.0625','0','0','2500';'AMP_Voltage_Signal','40','16','LE','unsigned','Standard','0','0.0625','-2000','-2000','2000'}
      settings: SourceProductBaseCode=ME,XP,VN  DataFormat=CANdb specified signals
  CAN_Msg : Subsystem
  CAN_Msg1 : Subsystem
  CAN_Msg2 : Subsystem
  CAN_Msg3 : Subsystem
  CAN_Msg_temp : Subsystem
  Constant : Constant  OutDataTypeStr=boolean
  Data Type Conversion{1..9} (9 alike) : DataTypeConversion  OutDataTypeStr=uint32
  FCAN_Transfer_Status1 : mbd_s32k1xx_ec_toolbox/Communication Blocks/CAN Blocks/FCAN_Transfer_Status  can_instance=1  can_mb_idx=17
  FCAN_Transfer_Status2 : mbd_s32k1xx_ec_toolbox/Communication Blocks/CAN Blocks/FCAN_Transfer_Status  can_instance=1  can_mb_idx=18
  FCAN_Transfer_Status3 : mbd_s32k1xx_ec_toolbox/Communication Blocks/CAN Blocks/FCAN_Transfer_Status  can_instance=1  can_mb_idx=16
  FCAN_Transfer_Status4 : mbd_s32k1xx_ec_toolbox/Communication Blocks/CAN Blocks/FCAN_Transfer_Status  can_instance=1  can_mb_idx=21
  FCAN_Transfer_Status5 : mbd_s32k1xx_ec_toolbox/Communication Blocks/CAN Blocks/FCAN_Transfer_Status  can_instance=1  can_mb_idx=20
  FCAN_Transfer_Status6 : mbd_s32k1xx_ec_toolbox/Communication Blocks/CAN Blocks/FCAN_Transfer_Status  can_instance=1  can_mb_idx=22
  FCAN_Transfer_Status7 : mbd_s32k1xx_ec_toolbox/Communication Blocks/CAN Blocks/FCAN_Transfer_Status  can_instance=1  can_mb_idx=19
  If{1..5,7..8} (7 alike) : If  NumInputs=2  IfExpression=u1 == 0 & u2 == 1  ShowElse=off
  MtrSts : Subsystem
  MtrSts1 : Subsystem
  PsngrWndwCntDetect : Subsystem
  RLWndwCntDetect : Subsystem
  RRWndwCntDetect : Subsystem
  Trigger : Stateflow chart  Commented=on  TreatAsAtomicUnit=on
  wires:
  If4/1 -> CAN_Msg1/Action
  If8/1 -> CAN_Msg/Action
  CAN Pack1/1 -> CAN_Msg/1(CAN_Msg)
  If2/1 -> CAN_Msg2/Action
  If5/1 -> CAN_Msg3/Action
  CAN Pack4/1 -> CAN_Msg1/1(CAN_Msg)
  CAN Pack2/1 -> CAN_Msg2/1(CAN_Msg)
  CAN Pack3/1 -> CAN_Msg3/1(CAN_Msg)
  HALL_2B_Freq_Count/1 -> CAN Pack5/6
  CAN Pack5/1 -> MtrSts/1(CAN_Msg)
  AmpBoard_PRV_CAN_Msg_TX1_CRC/1 -> CAN Pack5/2
  AmpBoard_PRV_CAN_Msg_TX1_Alive/1 -> CAN Pack5/1
  If7/1 -> MtrSts/Action
  HALL_1B_Freq_Count/1 -> CAN Pack5/4
  HALL_2A_Freq_Count/1 -> CAN Pack5/5
  HALL_1A_Freq_Count/1 -> CAN Pack5/3
  HALL_3A_Freq_Count/1 -> CAN Pack6/3
  HALL_4A_Freq_Count/1 -> CAN Pack6/5
  HALL_3B_Freq_Count/1 -> CAN Pack6/4
  If3/1 -> MtrSts1/Action
  AmpBoard_PRV_CAN_Msg_TX1B_Alive/1 -> CAN Pack6/1
  AmpBoard_PRV_CAN_Msg_TX1B_CRC/1 -> CAN Pack6/2
  CAN Pack6/1 -> MtrSts1/1(CAN_Msg)
  HALL_4B_Freq_Count/1 -> CAN Pack6/6
  AmpBoard_PRV_CAN_Msg_TX2_CRC/1 -> CAN Pack2/1
  AmpBoard_PRV_CAN_Msg_TX2_Alive/1 -> CAN Pack2/2
  AmpBoard_PRV_CAN_Msg_TX3B_Alive/1 -> CAN Pack4/4
  AmpBoard_PRV_CAN_Msg_TX3B_CRC/1 -> CAN Pack4/5
  An_In6/1 -> CAN Pack4/1
  An_In8/1 -> CAN Pack4/3
  An_In7/1 -> CAN Pack4/2
  An_In9/1 -> CAN Pack3/1
  An_In10/1 -> CAN Pack3/2
  AmpBoard_PRV_CAN_Msg_TX3C_Alive/1 -> CAN Pack3/5
  AmpBoard_PRV_CAN_Msg_TX3C_CRC/1 -> CAN Pack3/6
  An_In11/1 -> CAN Pack3/3
  An_In12/1 -> CAN Pack3/4
  AmpBoard_PRV_CAN_Msg_TX3_Alive/1 -> CAN Pack1/1
  AmpBoard_PRV_CAN_Msg_TX3_CRC/1 -> CAN Pack1/2
  Data Type Conversion1/1 -> CAN Pack1/6
  Data Type Conversion3/1 -> CAN Pack1/3
  Data Type Conversion2/1 -> CAN Pack4/6
  OsmMemoryAzimuthLeHa/1 -> CAN Pack1/4
  OsmMemoryElevationLeHa/1 -> CAN Pack1/5
  AB_ZC_ChildLockStatus/1 -> Data Type Conversion4/1
  DIGI_IN2/1 -> Data Type Conversion5/1
  DIGI_IN3/1 -> Data Type Conversion6/1
  DIGI_IN4/1 -> Data Type Conversion7/1
  DIGI_IN5/1 -> Data Type Conversion8/1
  DIGI_IN6/1 -> Data Type Conversion9/1
  DIGI_IN7/1 -> CAN Pack2/9
  DIGI_IN8/1 -> CAN Pack2/10
  DIGI_IN9/1 -> CAN Pack2/11
  DIGI_IN10/1 -> CAN Pack2/12
  Data Type Conversion4/1 -> CAN Pack2/3
  Data Type Conversion6/1 -> CAN Pack2/5
  Data Type Conversion8/1 -> CAN Pack2/7
  Data Type Conversion9/1 -> CAN Pack2/8
  Data Type Conversion5/1 -> CAN Pack2/4
  Data Type Conversion7/1 -> CAN Pack2/6
  If1/1 -> CAN_Msg_temp/Action
  AMP_Voltage_SIgnal/1 -> CAN Pack7/3
  CAN Pack7/1 -> CAN_Msg_temp/1(CAN_Msg)
  AMP_Status/1 -> CAN Pack7/1
  AMP_Temperature_Signal/1 -> CAN Pack7/2
  AB_ZC_PsngrWindowCommand/1 -> PsngrWndwCntDetect/1(SwitchCount)
  AB_ZC_RearRightWindowCommand/1 -> RRWndwCntDetect/1(SwitchCount)
  AB_ZC_RearLeftWindowCommand/1 -> RLWndwCntDetect/1(SwitchCount)
  [bool_TX] -> If8/2
  FCAN_Transfer_Status3/1 -> If8/1
  FCAN_Transfer_Status1/1 -> If4/1
  [bool_TX] -> If4/2
  [bool_TX] -> If2/2
  FCAN_Transfer_Status2/1 -> If2/1
  FCAN_Transfer_Status7/1 -> If1/1
  [bool_TX] -> If1/2
  [bool_TX] -> If7/2
  FCAN_Transfer_Status5/1 -> If7/1
  [bool_TX] -> If5/2
  FCAN_Transfer_Status4/1 -> If5/1
  [bool_TX] -> If3/2
  FCAN_Transfer_Status6/1 -> If3/1
  PsngrWndwCntDetect/1(AvgCount) -> Data Type Conversion3/1
  RRWndwCntDetect/1(AvgCount) -> Data Type Conversion1/1
  RLWndwCntDetect/1(AvgCount) -> Data Type Conversion2/1
  Constant/1 -> [bool_TX]

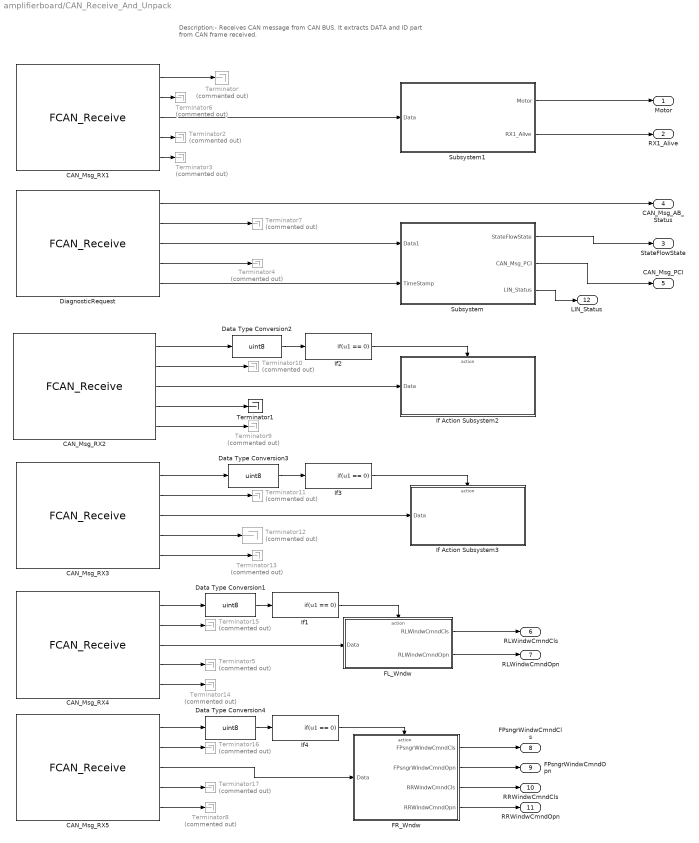
== system amplifierboard/CAN_Receive_And_Unpack ==
  note: Description:- Receives CAN message from CAN BUS. It extracts DATA and ID part from CAN frame received.
  CAN_Msg_RX1 : mbd_s32k1xx_ec_toolbox/Communication Blocks/CAN Blocks/FCAN_Receive  can_instance=1  can_mode=Blocking  can_timeout_ms=1000  can_mb_idx=1  can_mb_init=Once  show_id_input=off  can_extended_id=off  can_is_remote=off  can_id=2  can_msg_mask=FF  show_adv_opts=on  can_use_rxfifo=off  can_fd_enable=off
  CAN_Msg_RX2 : mbd_s32k1xx_ec_toolbox/Communication Blocks/CAN Blocks/FCAN_Receive  can_instance=1  can_mode=Blocking  can_timeout_ms=5  can_mb_idx=4  can_mb_init=Once  show_id_input=off  can_extended_id=off  can_is_remote=off  can_id=3  can_msg_mask=3  show_adv_opts=on  can_use_rxfifo=off  can_fd_enable=off
  CAN_Msg_RX3 : mbd_s32k1xx_ec_toolbox/Communication Blocks/CAN Blocks/FCAN_Receive  can_instance=1  can_mode=Blocking  can_timeout_ms=5  can_mb_idx=3  can_mb_init=Once  show_id_input=off  can_extended_id=off  can_is_remote=off  can_id=4  can_msg_mask=4  show_adv_opts=on  can_use_rxfifo=off  can_fd_enable=off
  CAN_Msg_RX4 : mbd_s32k1xx_ec_toolbox/Communication Blocks/CAN Blocks/FCAN_Receive  can_instance=1  can_mode=Blocking  can_timeout_ms=1000  can_mb_idx=5  can_mb_init=Once  show_id_input=off  can_extended_id=off  can_is_remote=off  can_id=110  can_msg_mask=FF  show_adv_opts=on  can_use_rxfifo=off  can_fd_enable=off
  CAN_Msg_RX5 : mbd_s32k1xx_ec_toolbox/Communication Blocks/CAN Blocks/FCAN_Receive  can_instance=1  can_mode=Blocking  can_timeout_ms=1000  can_mb_idx=6  can_mb_init=Once  show_id_input=off  can_extended_id=off  can_is_remote=off  can_id=110  can_msg_mask=FF  show_adv_opts=on  can_use_rxfifo=off  can_fd_enable=off
  Data Type Conversion{1..4} (4 alike) : DataTypeConversion  OutDataTypeStr=uint8
  DiagnosticRequest : mbd_s32k1xx_ec_toolbox/Communication Blocks/CAN Blocks/FCAN_Receive  can_instance=1  can_mode=Blocking  can_timeout_ms=5  can_mb_idx=0  can_mb_init=Once  show_id_input=off  can_extended_id=off  can_is_remote=off  can_id=AB  can_msg_mask=FF  show_adv_opts=on  can_use_rxfifo=off  can_fd_enable=off
  FL_Wndw : Subsystem  TreatAsAtomicUnit=on
  FR_Wndw : Subsystem  TreatAsAtomicUnit=on
  If Action Subsystem2 : Subsystem  TreatAsAtomicUnit=on
  If Action Subsystem3 : Subsystem  TreatAsAtomicUnit=on
  If{1..4} (4 alike) : If  IfExpression=u1 == 0  ShowElse=off
  Subsystem : Subsystem
  Subsystem1 : Subsystem
  Terminator{,2..17} (17 alike) : Terminator  Commented=on
  Terminator1 : Terminator
  Motor : Outport
  RX1_Alive : Outport  Port=2
  StateFlowState : Outport  Port=3
  CAN_Msg_AB_Status : Outport  Port=4
  CAN_Msg_PCI : Outport  Port=5
  RLWindwCmndCls : Outport  Port=6
  RLWindwCmndOpn : Outport  Port=7
  FPsngrWindwCmndCls : Outport  Port=8
  FPsngrWindwCmndOpn : Outport  Port=9
  RRWindwCmndCls : Outport  Port=10
  RRWindwCmndOpn : Outport  Port=11
  LIN_Status : Outport  Port=12
  wires:
  CAN_Msg_RX1/4 -> Terminator2/1
  CAN_Msg_RX1/5 -> Terminator3/1
  CAN_Msg_RX1/1 -> Terminator/1
  DiagnosticRequest/1 -> CAN_Msg_AB_Status/1
  DiagnosticRequest/5 -> Subsystem/2(TimeStamp)
  DiagnosticRequest/4 -> Terminator4/1
  DiagnosticRequest/3 -> Subsystem/1(Data1)
  If2/1 -> If Action Subsystem2/Action
  CAN_Msg_RX2/1 -> Data Type Conversion2/1
  CAN_Msg_RX2/5 -> Terminator9/1
  CAN_Msg_RX2/3 -> If Action Subsystem2/1(Data)
  CAN_Msg_RX2/4 -> Terminator1/1
  Data Type Conversion2/1 -> If2/1
  CAN_Msg_RX3/1 -> Data Type Conversion3/1
  Data Type Conversion3/1 -> If3/1
  CAN_Msg_RX3/5 -> Terminator13/1
  If3/1 -> If Action Subsystem3/Action
  CAN_Msg_RX3/3 -> If Action Subsystem3/1(Data)
  CAN_Msg_RX3/4 -> Terminator12/1
  Subsystem/1(StateFlowState) -> StateFlowState/1
  CAN_Msg_RX1/2 -> Terminator6/1
  DiagnosticRequest/2 -> Terminator7/1
  CAN_Msg_RX2/2 -> Terminator10/1
  CAN_Msg_RX3/2 -> Terminator11/1
  Subsystem/2(CAN_Msg_PCI) -> CAN_Msg_PCI/1
  CAN_Msg_RX1/3 -> Subsystem1/1(Data)
  Subsystem1/1(Motor) -> Motor/1
  Subsystem1/2(RX1_Alive) -> RX1_Alive/1
  CAN_Msg_RX4/5 -> Terminator14/1
  If1/1 -> FL_Wndw/Action
  Data Type Conversion1/1 -> If1/1
  FL_Wndw/1(RLWindwCmndCls) -> RLWindwCmndCls/1
  CAN_Msg_RX4/4 -> Terminator5/1
  CAN_Msg_RX4/1 -> Data Type Conversion1/1
  FL_Wndw/2(RLWindwCmndOpn) -> RLWindwCmndOpn/1
  CAN_Msg_RX4/3 -> FL_Wndw/1(Data)
  CAN_Msg_RX4/2 -> Terminator15/1
  If4/1 -> FR_Wndw/Action
  CAN_Msg_RX5/2 -> Terminator16/1
  CAN_Msg_RX5/4 -> Terminator17/1
  Data Type Conversion4/1 -> If4/1
  CAN_Msg_RX5/1 -> Data Type Conversion4/1
  CAN_Msg_RX5/3 -> FR_Wndw/1(Data)
  CAN_Msg_RX5/5 -> Terminator8/1
  FR_Wndw/3(RRWindwCmndCls) -> RRWindwCmndCls/1
  FR_Wndw/4(RRWindwCmndOpn) -> RRWindwCmndOpn/1
  FR_Wndw/2(FPsngrWindwCmndOpn) -> FPsngrWindwCmndOpn/1
  FR_Wndw/1(FPsngrWindwCmndCls) -> FPsngrWindwCmndCls/1
  Subsystem/3(LIN_Status) -> LIN_Status/1

== system amplifierboard/Digital_Input_Capture ==
  note: Description:- All Digital inputs(4) and SPARE inputs(3)are captured through digital GPIO block.Switch input capture debounce time is 50ms.
  AB_ZC_ChildLockStatus_In : mbd_s32k1xx_ec_toolbox/GPIO Blocks/Digital_Input  gpio_pin=PTE13: [PTE13 | Port E I/O]  pull_resistor=None  passive_filter=off
  Constant : Constant  Value=[0 0 0 0 0 0 0]  OutDataTypeStr=uint8
  Debounce1 : Subsystem
  Demux : Demux  Outputs=7
  Down_SwitchSts_In : mbd_s32k1xx_ec_toolbox/GPIO Blocks/Digital_Input  gpio_pin=PTC8: [PTC8 | Port C I/O]  pull_resistor=None  passive_filter=off
  FoldUnfold_SwitchSts_In : mbd_s32k1xx_ec_toolbox/GPIO Blocks/Digital_Input  gpio_pin=PTC2: [PTC2 | Port C I/O]  pull_resistor=None  passive_filter=off
  InvChldLck : Subsystem
  Left_SwitchSts_In : mbd_s32k1xx_ec_toolbox/GPIO Blocks/Digital_Input  gpio_pin=PTE1: [PTE1 | Port E I/O]  pull_resistor=None  passive_filter=off
  Logical Operator : Logic  Operator=OR  Inputs=7  AllPortsSameDT=off  OutDataTypeStr=boolean
  Mux1 : Mux  Inputs=7
      settings: DisplayOption=signals
  Right_SwitchSts_In : mbd_s32k1xx_ec_toolbox/GPIO Blocks/Digital_Input  gpio_pin=PTE14: [PTE14 | Port E I/O]  pull_resistor=None  passive_filter=off
  SPARE_IN3 : mbd_s32k1xx_ec_toolbox/GPIO Blocks/Digital_Input  gpio_pin=PTD2: [PTD2 | Port D I/O]  pull_resistor=None  passive_filter=off
  Switch : Switch  Criteria=u2 > Threshold
  Up_SwitchSts_In : mbd_s32k1xx_ec_toolbox/GPIO Blocks/Digital_Input  gpio_pin=PTA14: [PTA14 | Port A I/O]  pull_resistor=None  passive_filter=off
  AB_ZC_ChildLockStatus : Outport
  FoldUnfold_SwitchSts : Outport  Port=2
  Left_SwitchSts : Outport  Port=3
  Right_SwitchSts : Outport  Port=4
  UP_SwitchSts : Outport  Port=5
  Down_SwitchSts : Outport  Port=6
  SPARE_In3 : Outport  Port=7
  wires:
  FoldUnfold_SwitchSts_In/1 -> Logical Operator/2, Mux1/2
  Debounce1/1(Out1) -> Switch/2
  Left_SwitchSts_In/1 -> Logical Operator/3, Mux1/3
  Constant/1 -> Switch/3
  Right_SwitchSts_In/1 -> Logical Operator/4, Mux1/4
  Switch/1 -> Demux/1
  Logical Operator/1 -> Debounce1/1(In1)
  AB_ZC_ChildLockStatus_In/1 -> Logical Operator/1, Mux1/1
  Mux1/1 -> Switch/1
  Demux/1 -> InvChldLck/1(In)
  Up_SwitchSts_In/1 -> Logical Operator/5, Mux1/5
  Down_SwitchSts_In/1 -> Logical Operator/6, Mux1/6
  SPARE_IN3/1 -> Logical Operator/7, Mux1/7
  Demux/7 -> SPARE_In3/1
  Demux/3 -> Left_SwitchSts/1
  Demux/2 -> FoldUnfold_SwitchSts/1
  Demux/4 -> Right_SwitchSts/1
  Demux/5 -> UP_SwitchSts/1
  Demux/6 -> Down_SwitchSts/1
  InvChldLck/1(ChildLock) -> AB_ZC_ChildLockStatus/1

== system amplifierboard/HALL_Input_Capture ==
  note: HALL Input Capture
      | Version :-1.0.0
      | Sample Rate :-10ms
      | Description:- All HALL sensors input will be captured here and corrosponding hall count is calculated(HE1 tp HE8)
  Demux : Demux  Outputs=8
  HEEvents : Subsystem
  Hall_Count_Calculation : Stateflow chart  TreatAsAtomicUnit=on
  HALL_1A_Freq_Count : Outport
  HALL_1B_Freq_Count : Outport  Port=2
  HALL_2A_Freq_Count : Outport  Port=3
  HALL_2B_Freq_Count : Outport  Port=4
  HALL_3A_Freq_Count : Outport  Port=5
  HALL_3B_Freq_Count : Outport  Port=6
  HALL_4A_Freq_Count : Outport  Port=7
  HALL_4B_Freq_Count : Outport  Port=8
  wires:
  Demux/7 -> HALL_4A_Freq_Count/1
  Demux/8 -> HALL_4B_Freq_Count/1
  Demux/5 -> HALL_3A_Freq_Count/1
  Hall_Count_Calculation/1(MotorPosCount) -> Demux/1
  Demux/2 -> HALL_1B_Freq_Count/1
  HEEvents/1(Events) -> Hall_Count_Calculation/Trigger
  Demux/4 -> HALL_2B_Freq_Count/1
  Demux/1 -> HALL_1A_Freq_Count/1
  Demux/3 -> HALL_2A_Freq_Count/1
  Demux/6 -> HALL_3B_Freq_Count/1
